simulink library "Damper_LeftRight_AsymmetricNonlinear"  (R2026a)
settings: Solver=VariableStepAuto
libraries: Damper_Nonlinear x2, fl_lib x2
Description:
  | Component of Simscape Vehicle Templates Library
  | 
  | Copyright 2018-2024 The MathWorks, Inc.
settings Model: Creator=smiller  LastModifiedBy=smiller

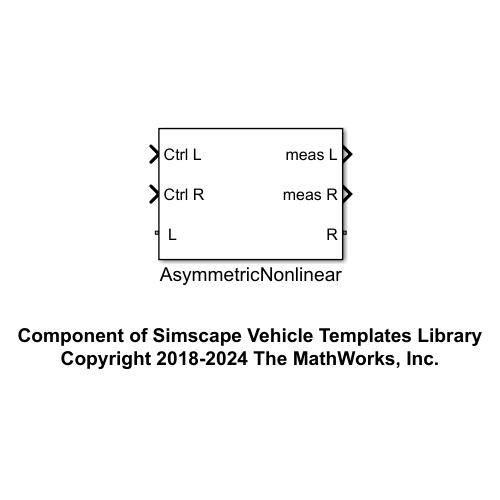
[thumbnail: Simulink's stored preview of the top-level diagram]
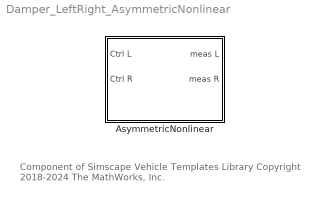
== system Damper_LeftRight_AsymmetricNonlinear ==
  note: Component of Simscape Vehicle Templates Library
      | Copyright 2018-2024 The MathWorks, Inc.
  AsymmetricNonlinear : Subsystem  VariantControl=Linear  mask(Asymmetric Nonlinear Dampers){}
      mask help: Dampers with independent hardpoint parameterization for left and right sides. For damper connections in suspensions that may be asymmetric at design position, such as Panhard rod suspensions.

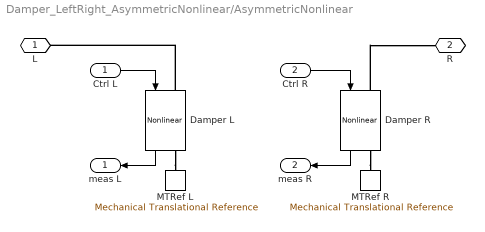
== system Damper_LeftRight_AsymmetricNonlinear/AsymmetricNonlinear ==
  Ctrl L : Inport
  Ctrl R : Inport  Port=2
  Damper L : Damper_Nonlinear/Nonlinear  VariantControl=Nonlinear  velocity_vector=Damper.Damping.vDamperL.Value  force_vector=Damper.Damping.fDamperL.Value  hp_dpr_top=Damper.Damping.sTopL.Value  hp_dpr_bot=Damper.Damping.sBottomL.Value  bs_lim_upper=Damper.Endstop.xMax.Value  bs_lim_lower=Damper.Endstop.xMin.Value  bs_k_upper=Damper.Endstop.KxMax.Value  bs_k_lower=Damper.Endstop.KxMin.Value  bs_b_upper=Damper.Endstop.dxMax.Value  bs_b_lower=Damper.Endstop.dxMin.Value  bs_region=Damper.Endstop.xTransition.Value
  Damper R : Damper_Nonlinear/Nonlinear  VariantControl=Nonlinear  velocity_vector=Damper.Damping.vDamperR.Value  force_vector=Damper.Damping.fDamperR.Value  hp_dpr_top=Damper.Damping.sTopR.Value  hp_dpr_bot=Damper.Damping.sBottomR.Value  bs_lim_upper=Damper.Endstop.xMax.Value  bs_lim_lower=Damper.Endstop.xMin.Value  bs_k_upper=Damper.Endstop.KxMax.Value  bs_k_lower=Damper.Endstop.KxMin.Value  bs_b_upper=Damper.Endstop.dxMax.Value  bs_b_lower=Damper.Endstop.dxMin.Value  bs_region=Damper.Endstop.xTransition.Value
  MTRef L : fl_lib/Mechanical/Translational Elements/Mechanical Translational Reference
  MTRef R : fl_lib/Mechanical/Translational Elements/Mechanical Translational Reference
  " L" : PMIOPort  Side=Left
  " R" : PMIOPort  Port=2  Side=Right
  meas L : Outport  VectorParamsAs1DForOutWhenUnconnected=off
  meas R : Outport  Port=2  VectorParamsAs1DForOutWhenUnconnected=off
  wires:
  Damper L/1 -> meas L/1
  Ctrl L/1 -> Damper L/1
  Ctrl R/1 -> Damper R/1
  Damper R/1 -> meas R/1
  connections:
  Damper L/RConn1 -- MTRef L/LConn1
  Damper R/LConn1 -- " R"/RConn1
  Damper R/RConn1 -- MTRef R/LConn1
  Damper L/LConn1 -- " L"/RConn1
